simulink model "DS_CDMA1"  (Simulink 6.1)
settings: Solver=ode45  StartTime=0.0  StopTime=1  RelTol=1e-3
undefined symbols (not defined in the file or in its folder): magnitude
libraries: dspsigops x14, commdigbbndpm2 x3, commchan2 x2, dspstat3 x2, commseqgen2 x2, commrandsrc2 x1
settings Model: Creator=Hexingjian  LastModifiedBy=Administrator
settings OptimizationCC: InlineInvariantSignals=off
settings DebuggingCC: SignalResolutionControl=UseLocalSettings  MultiTaskDSMMsg=error

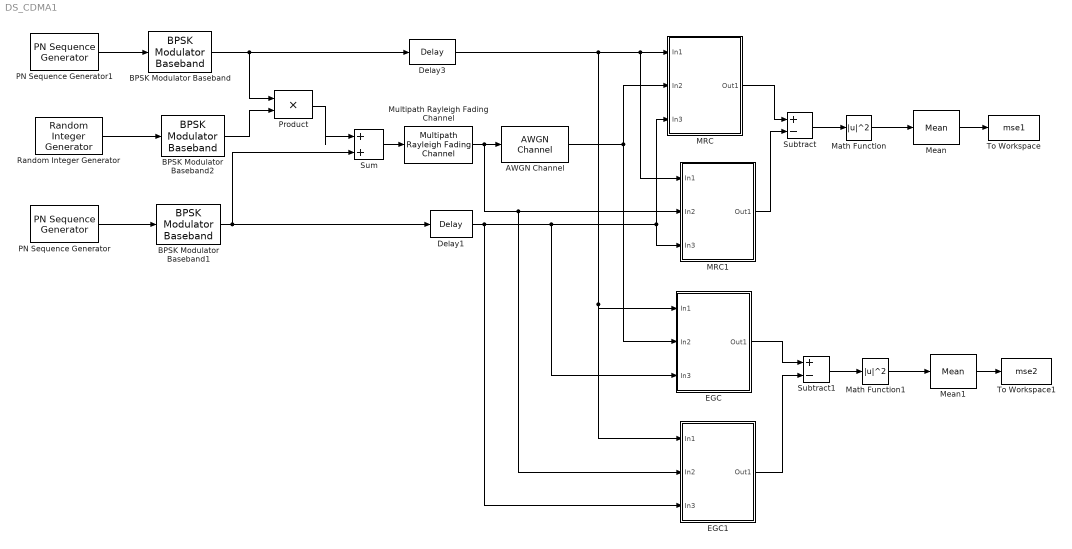
== system DS_CDMA1 ==
  AWGN Channel : commchan2/AWGN Channel  seed=67  noiseMode="Signal to noise ratio  (SNR)"  EbNodB=10  EsNodB=10  SNRdB=SNR  bitsPerSym=1  Ps=1  Tsym=1e-4/32  variance=1
  BPSK Modulator Baseband : commdigbbndpm2/BPSK Modulator Baseband  Ph=0  numSamp=1
  BPSK Modulator Baseband1 : commdigbbndpm2/BPSK Modulator Baseband  Ph=0  numSamp=1
  BPSK Modulator Baseband2 : commdigbbndpm2/BPSK Modulator Baseband  Ph=0  numSamp=1
  Delay1 : dspsigops/Delay  dly_unit=Samples  delay=32  ic_detail=off  dif_ic_for_ch=off  dif_ic_for_dly=off  ic=0  reset_popup=None
  Delay3 : dspsigops/Delay  dly_unit=Samples  delay=32  ic_detail=off  dif_ic_for_ch=off  dif_ic_for_dly=off  ic=0  reset_popup=None
  EGC : Subsystem
  EGC1 : Subsystem
  MRC : Subsystem
  MRC1 : Subsystem
  Math Function : Math  Operator=magnitude^2  SaturateOnIntegerOverflow=on
  Math Function1 : Math  Operator=magnitude^2  SaturateOnIntegerOverflow=on
  Mean : dspstat3/Mean  DialogController=dspDDGCreate  DialogControllerArgs=DataTag0  run=off  reset_popup=None  roundingMode=Floor  overflowMode=off
  Mean1 : dspstat3/Mean  DialogController=dspDDGCreate  DialogControllerArgs=DataTag1  run=off  reset_popup=None  roundingMode=Floor  overflowMode=off
  Multipath Rayleigh Fading Channel : commchan2/Multipath Rayleigh Fading Channel  Fd=100  simTs=1e-4/32  delayVec=[0 8e-4/32 16e-4/32]  gainVecdB=[0 -3 -6]  normGain=on  Seed=73
  PN Sequence Generator : commseqgen2/PN Sequence Generator  poly=[15 13 12 10 9 8 7 5 4 1 0]  ini_sta=[0 0 1 0 0 0 1 0 0 0 1 0 0 0 1]  shift=0  Ts=1e-4/32  frameBased=on  sampPerFrame=32  reset=off
  PN Sequence Generator1 : commseqgen2/PN Sequence Generator  poly=[15 14 10 7 6 2 0]  ini_sta=[1 0 0 0 1 0 0 0 1 0 0 0 1 0 0]  shift=0  Ts=1e-4/32  frameBased=on  sampPerFrame=32  reset=off
  Product : Product  SaturateOnIntegerOverflow=on
  Random Integer Generator : commrandsrc2/Random Integer Generator  mul=2  seed=37  Ts=1e-4  frameBased=on  sampPerFrame=1  orient=off
  Subtract : Sum  Inputs=+-  OutScaling=2^-10
  Subtract1 : Sum  Inputs=+-  OutScaling=2^-10
  Sum : Sum  Inputs=|++  SaturateOnIntegerOverflow=on
  To Workspace : ToWorkspace  VariableName=mse1  SampleTime=-1  SaveFormat=Array
  To Workspace1 : ToWorkspace  VariableName=mse2  SampleTime=-1  SaveFormat=Array
  wires:
  Random Integer Generator/1 -> BPSK Modulator Baseband2/1
  PN Sequence Generator1/1 -> BPSK Modulator Baseband/1
  PN Sequence Generator/1 -> BPSK Modulator Baseband1/1
  BPSK Modulator Baseband/1 -> Product/1, Delay3/1
  BPSK Modulator Baseband2/1 -> Product/2
  BPSK Modulator Baseband1/1 -> Sum/2, Delay1/1
  Product/1 -> Sum/1
  Sum/1 -> Multipath Rayleigh Fading Channel/1
  Multipath Rayleigh Fading Channel/1 -> AWGN Channel/1, MRC1/2(In2), EGC1/2(In2)
  AWGN Channel/1 -> MRC/2(In2), EGC/2(In2)
  Delay3/1 -> MRC/1(In1), MRC1/1(In1), EGC/1(In1), EGC1/1(In1)
  Delay1/1 -> EGC/3(In3), MRC/3(In3), MRC1/3(In3), EGC1/3(In3)
  Subtract/1 -> Math Function/1
  Math Function/1 -> Mean/1
  Mean/1 -> To Workspace/1
  MRC/1(Out1) -> Subtract/1
  MRC1/1(Out1) -> Subtract/2
  Subtract1/1 -> Math Function1/1
  Math Function1/1 -> Mean1/1
  Mean1/1 -> To Workspace1/1
  EGC/1(Out1) -> Subtract1/1
  EGC1/1(Out1) -> Subtract1/2

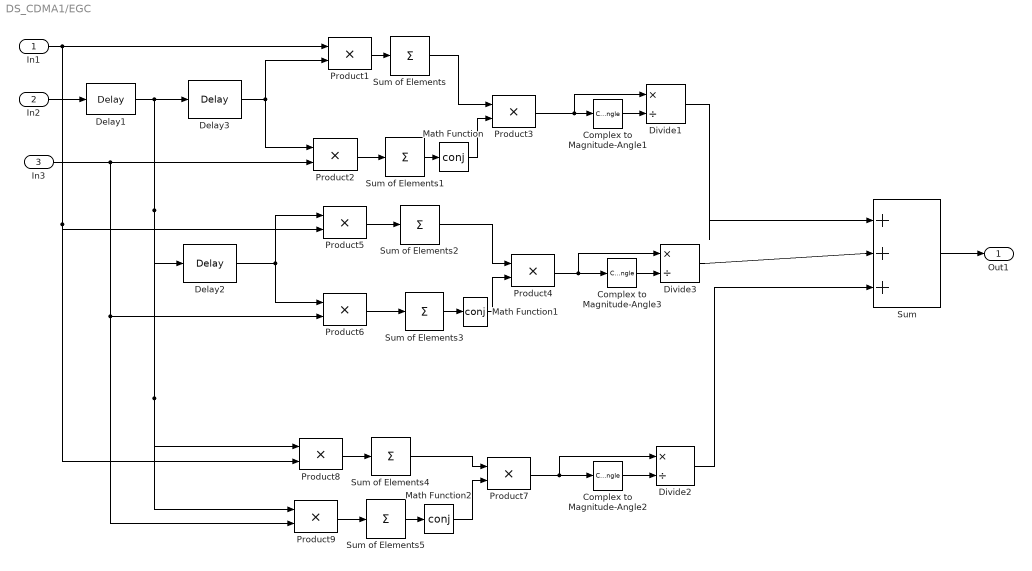
== system DS_CDMA1/EGC ==
  In1 : Inport  Port=1  LatchInput=off
  In2 : Inport  Port=2  LatchInput=off
  In3 : Inport  Port=3  LatchInput=off
  Complex to Magnitude-Angle1 : ComplexToMagnitudeAngle  Output=Magnitude
  Complex to Magnitude-Angle2 : ComplexToMagnitudeAngle  Output=Magnitude
  Complex to Magnitude-Angle3 : ComplexToMagnitudeAngle  Output=Magnitude
  Delay1 : dspsigops/Delay  dly_unit=Samples  delay=16  ic_detail=off  dif_ic_for_ch=off  dif_ic_for_dly=off  ic=0  reset_popup=None
  Delay2 : dspsigops/Delay  dly_unit=Samples  delay=8  ic_detail=off  dif_ic_for_ch=off  dif_ic_for_dly=off  ic=0  reset_popup=None
  Delay3 : dspsigops/Delay  dly_unit=Samples  delay=16  ic_detail=off  dif_ic_for_ch=off  dif_ic_for_dly=off  ic=0  reset_popup=None
  Divide1 : Product  Inputs=*/  OutScaling=2^-10
  Divide2 : Product  Inputs=*/  OutScaling=2^-10
  Divide3 : Product  Inputs=*/  OutScaling=2^-10
  Math Function : Math  Operator=conj  SaturateOnIntegerOverflow=on
  Math Function1 : Math  Operator=conj  SaturateOnIntegerOverflow=on
  Math Function2 : Math  Operator=conj  SaturateOnIntegerOverflow=on
  Product{1..9} (9 alike) : Product  SaturateOnIntegerOverflow=on
  Sum : Sum  Inputs=|+++  SaturateOnIntegerOverflow=on
  Sum of Elements{,1..5} (6 alike) : Sum  Inputs=+  OutScaling=2^-10
  Out1 : Outport
  wires:
  In2/1 -> Delay1/1
  Sum of Elements1/1 -> Math Function/1
  Product2/1 -> Sum of Elements1/1
  Sum of Elements/1 -> Product3/1
  Product1/1 -> Sum of Elements/1
  In1/1 -> Product1/1, Product8/2, Product5/2
  In3/1 -> Product2/2, Product9/2, Product6/2
  Math Function/1 -> Product3/2
  Sum/1 -> Out1/1
  Delay3/1 -> Product1/2, Product2/1
  Delay1/1 -> Delay3/1, Product9/1, Product8/1, Delay2/1
  Sum of Elements3/1 -> Math Function1/1
  Sum of Elements2/1 -> Product4/1
  Product6/1 -> Sum of Elements3/1
  Product5/1 -> Sum of Elements2/1
  Math Function1/1 -> Product4/2
  Product8/1 -> Sum of Elements4/1
  Product9/1 -> Sum of Elements5/1
  Sum of Elements4/1 -> Product7/1
  Sum of Elements5/1 -> Math Function2/1
  Math Function2/1 -> Product7/2
  Delay2/1 -> Product5/1, Product6/1
  Complex to Magnitude-Angle1/1 -> Divide1/2
  Product3/1 -> Complex to Magnitude-Angle1/1, Divide1/1
  Divide1/1 -> Sum/1
  Complex to Magnitude-Angle2/1 -> Divide2/2
  Product7/1 -> Complex to Magnitude-Angle2/1, Divide2/1
  Divide2/1 -> Sum/3
  Complex to Magnitude-Angle3/1 -> Divide3/2
  Product4/1 -> Complex to Magnitude-Angle3/1, Divide3/1
  Divide3/1 -> Sum/2

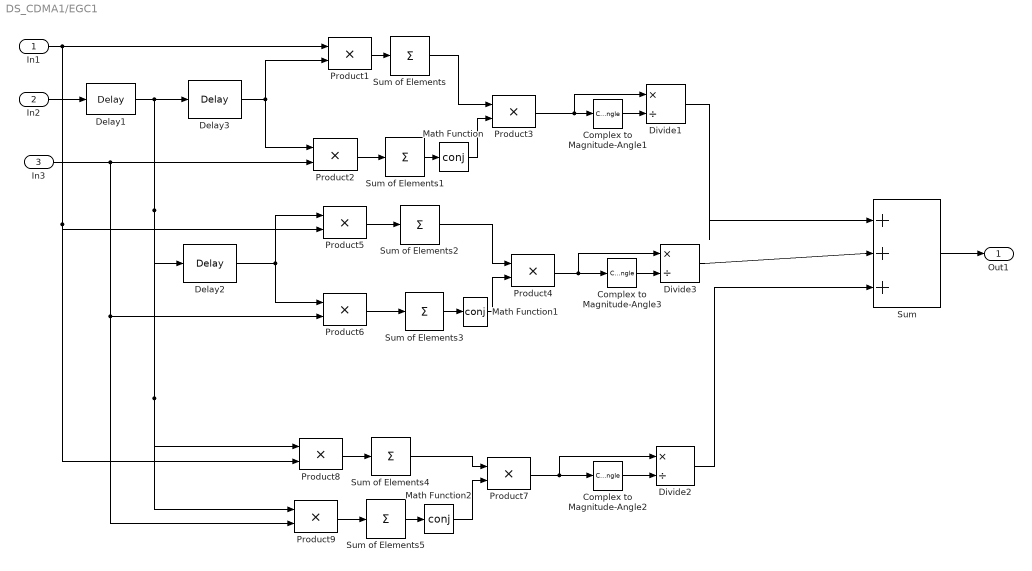
== system DS_CDMA1/EGC1 ==
  In1 : Inport  Port=1  LatchInput=off
  In2 : Inport  Port=2  LatchInput=off
  In3 : Inport  Port=3  LatchInput=off
  Complex to Magnitude-Angle1 : ComplexToMagnitudeAngle  Output=Magnitude
  Complex to Magnitude-Angle2 : ComplexToMagnitudeAngle  Output=Magnitude
  Complex to Magnitude-Angle3 : ComplexToMagnitudeAngle  Output=Magnitude
  Delay1 : dspsigops/Delay  dly_unit=Samples  delay=16  ic_detail=off  dif_ic_for_ch=off  dif_ic_for_dly=off  ic=0  reset_popup=None
  Delay2 : dspsigops/Delay  dly_unit=Samples  delay=8  ic_detail=off  dif_ic_for_ch=off  dif_ic_for_dly=off  ic=0  reset_popup=None
  Delay3 : dspsigops/Delay  dly_unit=Samples  delay=16  ic_detail=off  dif_ic_for_ch=off  dif_ic_for_dly=off  ic=0  reset_popup=None
  Divide1 : Product  Inputs=*/  OutScaling=2^-10
  Divide2 : Product  Inputs=*/  OutScaling=2^-10
  Divide3 : Product  Inputs=*/  OutScaling=2^-10
  Math Function : Math  Operator=conj  SaturateOnIntegerOverflow=on
  Math Function1 : Math  Operator=conj  SaturateOnIntegerOverflow=on
  Math Function2 : Math  Operator=conj  SaturateOnIntegerOverflow=on
  Product{1..9} (9 alike) : Product  SaturateOnIntegerOverflow=on
  Sum : Sum  Inputs=|+++  SaturateOnIntegerOverflow=on
  Sum of Elements{,1..5} (6 alike) : Sum  Inputs=+  OutScaling=2^-10
  Out1 : Outport
  wires:
  In2/1 -> Delay1/1
  Sum of Elements1/1 -> Math Function/1
  Product2/1 -> Sum of Elements1/1
  Sum of Elements/1 -> Product3/1
  Product1/1 -> Sum of Elements/1
  In1/1 -> Product1/1, Product8/2, Product5/2
  In3/1 -> Product2/2, Product9/2, Product6/2
  Math Function/1 -> Product3/2
  Sum/1 -> Out1/1
  Delay3/1 -> Product1/2, Product2/1
  Delay1/1 -> Delay3/1, Product9/1, Product8/1, Delay2/1
  Sum of Elements3/1 -> Math Function1/1
  Sum of Elements2/1 -> Product4/1
  Product6/1 -> Sum of Elements3/1
  Product5/1 -> Sum of Elements2/1
  Math Function1/1 -> Product4/2
  Product8/1 -> Sum of Elements4/1
  Product9/1 -> Sum of Elements5/1
  Sum of Elements4/1 -> Product7/1
  Sum of Elements5/1 -> Math Function2/1
  Math Function2/1 -> Product7/2
  Delay2/1 -> Product5/1, Product6/1
  Complex to Magnitude-Angle1/1 -> Divide1/2
  Product3/1 -> Complex to Magnitude-Angle1/1, Divide1/1
  Divide1/1 -> Sum/1
  Complex to Magnitude-Angle2/1 -> Divide2/2
  Product7/1 -> Complex to Magnitude-Angle2/1, Divide2/1
  Divide2/1 -> Sum/3
  Complex to Magnitude-Angle3/1 -> Divide3/2
  Product4/1 -> Complex to Magnitude-Angle3/1, Divide3/1
  Divide3/1 -> Sum/2

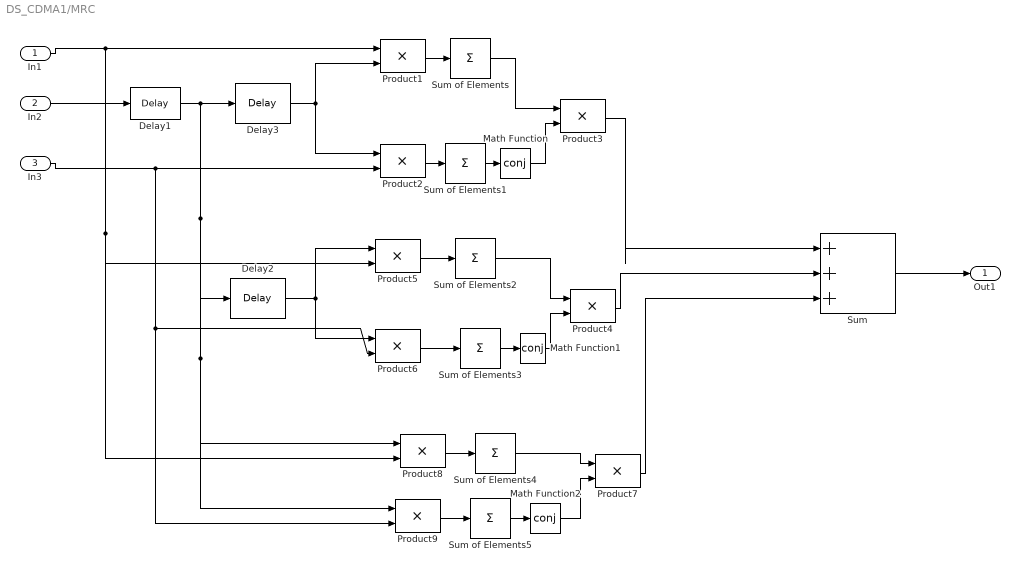
== system DS_CDMA1/MRC ==
  In1 : Inport  Port=1  LatchInput=off
  In2 : Inport  Port=2  LatchInput=off
  In3 : Inport  Port=3  LatchInput=off
  Delay1 : dspsigops/Delay  dly_unit=Samples  delay=16  ic_detail=off  dif_ic_for_ch=off  dif_ic_for_dly=off  ic=0  reset_popup=None
  Delay2 : dspsigops/Delay  dly_unit=Samples  delay=8  ic_detail=off  dif_ic_for_ch=off  dif_ic_for_dly=off  ic=0  reset_popup=None
  Delay3 : dspsigops/Delay  dly_unit=Samples  delay=16  ic_detail=off  dif_ic_for_ch=off  dif_ic_for_dly=off  ic=0  reset_popup=None
  Math Function : Math  Operator=conj  SaturateOnIntegerOverflow=on
  Math Function1 : Math  Operator=conj  SaturateOnIntegerOverflow=on
  Math Function2 : Math  Operator=conj  SaturateOnIntegerOverflow=on
  Product{1..9} (9 alike) : Product  SaturateOnIntegerOverflow=on
  Sum : Sum  Inputs=|+++  SaturateOnIntegerOverflow=on
  Sum of Elements{,1..5} (6 alike) : Sum  Inputs=+  OutScaling=2^-10
  Out1 : Outport
  wires:
  In2/1 -> Delay1/1
  Sum of Elements1/1 -> Math Function/1
  Product2/1 -> Sum of Elements1/1
  Sum of Elements/1 -> Product3/1
  Product1/1 -> Sum of Elements/1
  In1/1 -> Product1/1, Product8/2, Product5/2
  In3/1 -> Product2/2, Product9/2, Product6/2
  Product3/1 -> Sum/1
  Math Function/1 -> Product3/2
  Sum/1 -> Out1/1
  Delay3/1 -> Product1/2, Product2/1
  Delay1/1 -> Delay3/1, Product9/1, Product8/1, Delay2/1
  Sum of Elements3/1 -> Math Function1/1
  Sum of Elements2/1 -> Product4/1
  Product6/1 -> Sum of Elements3/1
  Product5/1 -> Sum of Elements2/1
  Product4/1 -> Sum/2
  Math Function1/1 -> Product4/2
  Product8/1 -> Sum of Elements4/1
  Product9/1 -> Sum of Elements5/1
  Sum of Elements4/1 -> Product7/1
  Sum of Elements5/1 -> Math Function2/1
  Math Function2/1 -> Product7/2
  Product7/1 -> Sum/3
  Delay2/1 -> Product5/1, Product6/1

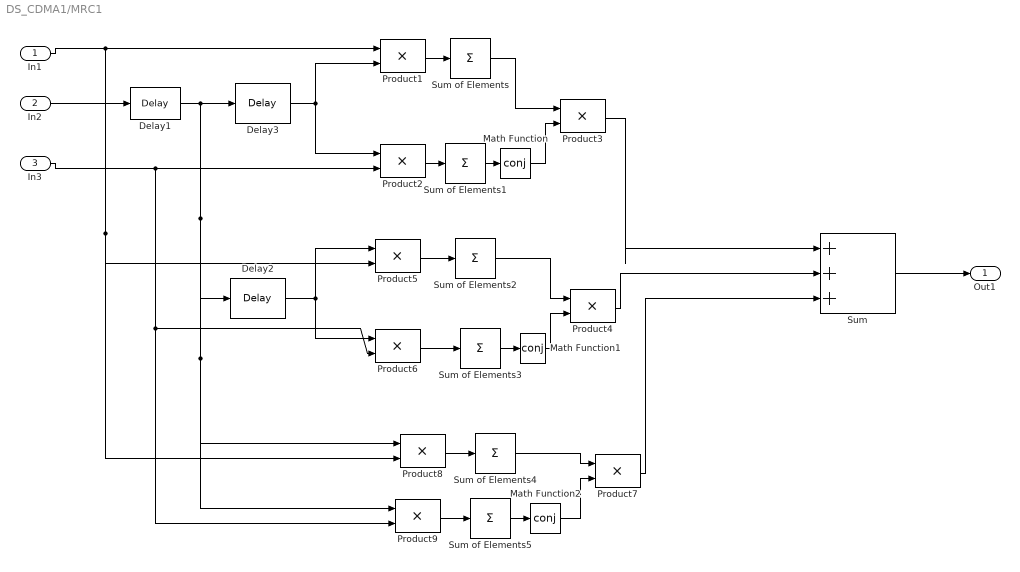
== system DS_CDMA1/MRC1 ==
  In1 : Inport  Port=1  LatchInput=off
  In2 : Inport  Port=2  LatchInput=off
  In3 : Inport  Port=3  LatchInput=off
  Delay1 : dspsigops/Delay  dly_unit=Samples  delay=16  ic_detail=off  dif_ic_for_ch=off  dif_ic_for_dly=off  ic=0  reset_popup=None
  Delay2 : dspsigops/Delay  dly_unit=Samples  delay=8  ic_detail=off  dif_ic_for_ch=off  dif_ic_for_dly=off  ic=0  reset_popup=None
  Delay3 : dspsigops/Delay  dly_unit=Samples  delay=16  ic_detail=off  dif_ic_for_ch=off  dif_ic_for_dly=off  ic=0  reset_popup=None
  Math Function : Math  Operator=conj  SaturateOnIntegerOverflow=on
  Math Function1 : Math  Operator=conj  SaturateOnIntegerOverflow=on
  Math Function2 : Math  Operator=conj  SaturateOnIntegerOverflow=on
  Product{1..9} (9 alike) : Product  SaturateOnIntegerOverflow=on
  Sum : Sum  Inputs=|+++  SaturateOnIntegerOverflow=on
  Sum of Elements{,1..5} (6 alike) : Sum  Inputs=+  OutScaling=2^-10
  Out1 : Outport
  wires:
  In2/1 -> Delay1/1
  Sum of Elements1/1 -> Math Function/1
  Product2/1 -> Sum of Elements1/1
  Sum of Elements/1 -> Product3/1
  Product1/1 -> Sum of Elements/1
  In1/1 -> Product1/1, Product8/2, Product5/2
  In3/1 -> Product2/2, Product9/2, Product6/2
  Product3/1 -> Sum/1
  Math Function/1 -> Product3/2
  Sum/1 -> Out1/1
  Delay3/1 -> Product1/2, Product2/1
  Delay1/1 -> Delay3/1, Product9/1, Product8/1, Delay2/1
  Sum of Elements3/1 -> Math Function1/1
  Sum of Elements2/1 -> Product4/1
  Product6/1 -> Sum of Elements3/1
  Product5/1 -> Sum of Elements2/1
  Product4/1 -> Sum/2
  Math Function1/1 -> Product4/2
  Product8/1 -> Sum of Elements4/1
  Product9/1 -> Sum of Elements5/1
  Sum of Elements4/1 -> Product7/1
  Sum of Elements5/1 -> Math Function2/1
  Math Function2/1 -> Product7/2
  Product7/1 -> Sum/3
  Delay2/1 -> Product5/1, Product6/1
